simulink model "sgMdl_OPCUA_Security"  (R2024b)
settings: Solver=FixedStepAuto  StartTime=0.0  StopTime=inf  RelTol=1e-3  EnableMultiTasking=on
undefined symbols (not defined in the file): filesep, Ts
libraries: speedgoatlib_opcua x25, simulink x10
Description:
  | OPC UA Security
settings Model: sg_rtwmakecfg_data=_sg_IO75X_v1_2_0__sg_netxLib_MSVC140_  ModifiedByFormat=Speedgoat  Creator=Speedgoat  LastModifiedBy=Speedgoat
settings SolverCC: ConcurrentTasks=on  AlgebraicLoopSolver=TrustRegion  PositivePriorityOrder=on  AutoInsertRateTranBlk=on  InsertRTBMode=Never (minimum delay)  MaxZcPerStep=1
settings DataIOCC: LimitDataPoints=on  SaveFormat=StructureWithTime  ReturnWorkspaceOutputs=off
settings OptimizationCC: BlockReduction=off  BooleanDataType=off  OptimizeBlockIOStorage=off  BufferReuse=off  GlobalBufferReuse=off  ExpressionFolding=off  LocalBlockOutputs=off  OptimizeDataStoreBuffers=off  BusAssignmentInplaceUpdate=off
settings DebuggingCC: SaveWithParameterizedLinksMsg=none  UnderspecifiedInitializationDetection=Classic  MergeDetectMultiDrivingBlocksExec=none  SignalResolutionControl=TryResolveAllWithWarning  TasksWithSamePriorityMsg=none  ParameterOverflowMsg=warning  UnconnectedInputMsg=warning  UnconnectedOutputMsg=warning  UnconnectedLineMsg=warning  SFUnexpectedBacktrackingDiag=warning  SFNoUnconditionalDefaultTransitionDiag=warning  SFExecutionAtInitializationDiag=none  ArithmeticOperatorsInVariantConditions=warning
settings HardwareCC: ProdBitPerLong=64  ProdLongLongMode=on  ProdHWDeviceType=Intel->x86-64 (Linux 64)  TargetBitPerPointer=64  TargetBitPerSizeT=64  TargetBitPerPtrDiffT=64  TargetLongLongMode=on  TargetIntDivRoundTo=Zero  TargetEndianess=LittleEndian  TargetWordSize=64  TargetHWDeviceType=MATLAB Host
settings ModelReferenceCC: EnableRefExpFcnMdlSchedulingChecks=on  PropagateSignalLabelsOutOfModel=off
settings SFSimCC: SimUseLocalCustomCode=off  CustomCodeUndefinedFunction=UseInterfaceOnly
settings RTWCC: Description=Speedgoat Real-Time Target Machine  SystemTargetFile=speedgoat.tlc  TemplateMakefile=slrealtime_default_tmf  RetainRTWFile=on  RTWUseLocalCustomCode=off  Toolchain=Simulink Real-Time Toolchain  BuildConfiguration=Faster Runs  TargetLang=C++  GPUComputeCapability=3.5  DLArmComputeVersion=19.05
settings CodeAppCC: StateflowObjectComments=on
settings SimulinkRealTimeTargetCC: SubcomponentCodeInterfacePackaging=Reusable function  InstructionSetFMA=off  LogToMDFFile=off  SLRTFileLogMaxRuns=10
settings ConfigComp: CovMetricSettings=dw  CovSaveCumulativeToWorkspaceVar=on  CovSaveSingleToWorkspaceVar=on  CovExternalEMLEnable=off  CovBoundaryAbsTol=1.0e-5

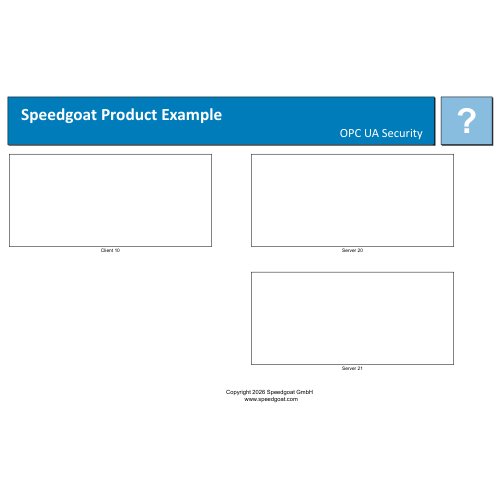
[thumbnail: Simulink's stored preview of the top-level diagram]
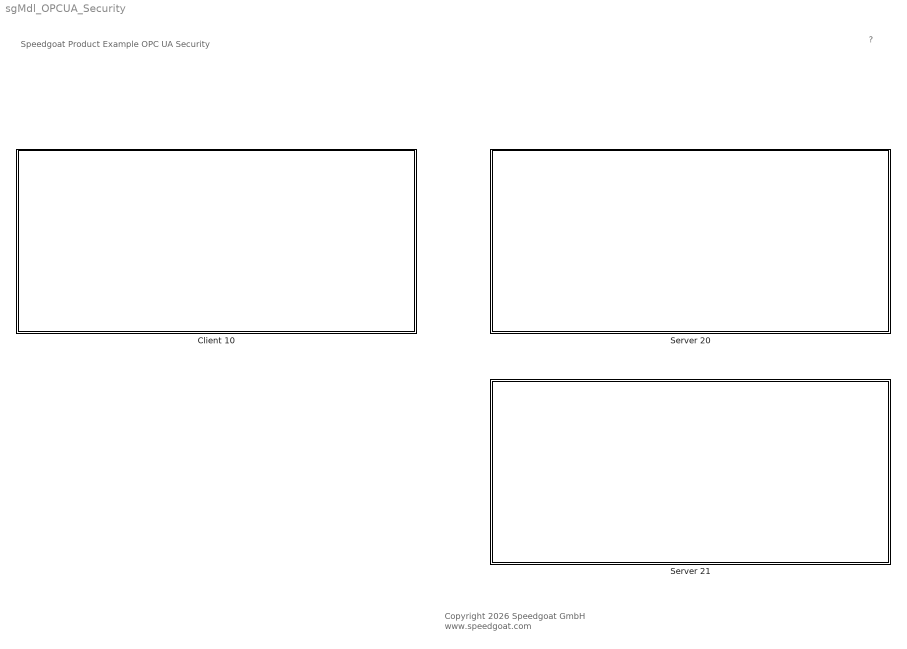
== system sgMdl_OPCUA_Security ==
  note: Speedgoat Product Example
      | OPC UA Security
  note: ?
  note: Copyright 2026 Speedgoat GmbH
      |  www.speedgoat.com
  Client 10 : Subsystem
  Server 20 : Subsystem
  Server 21 : Subsystem

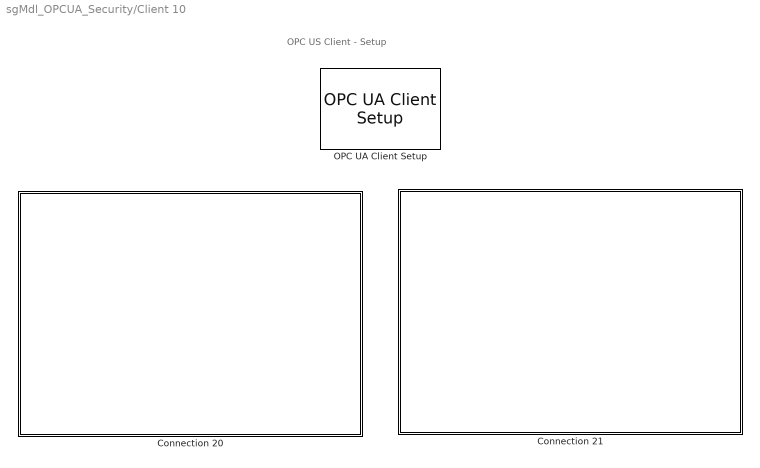
== system sgMdl_OPCUA_Security/Client 10 ==
  note: OPC US Client - Setup
  Connection 20 : Subsystem
  Connection 21 : Subsystem
  OPC UA Client Setup : speedgoatlib_opcua/Client/OPC UA Client Setup  ClientID=10  IpAddrStr=IP_Client_10
      settings: SourceProductName=OPC UA

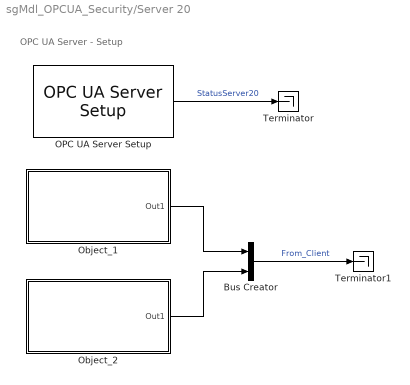
== system sgMdl_OPCUA_Security/Server 20 ==
  note: OPC UA Server - Setup
  Bus Creator : BusCreator  Inputs=2
  OPC UA Server Setup : speedgoatlib_opcua/Server/OPC UA Server Setup  ServerID=20  IpAddrStr=IP_Server_20  TcpPort=4840  NumSpaces=0  SampleTime=Ts  Endpoints={ 'None', 'on', 'None'; 'Basic128Rsa15', 'on', 'SignEncrypt'; 'Basic256', 'off', 'SignEncrypt'; 'Basic256Sha256', 'off', 'SignEncrypt'; 'Aes128_Sha256_RsaOaep', 'on', 'SignEncrypt' }  AnonymousToken=on  UsernameToken=on  Certificate=fullfile(pwd, filesep, 'cert', filesep, 'sg_server1.der')  PrivateKey=fullfile(pwd, filesep, 'cert', filesep, 'sg_key.pem')  TrustList=''  Usernames="[\"user1\", \"user2\"]"  Passwords="[\"password1\", \"password2\"]"  AppUri='urn:sg:server1'
      settings: SourceProductName=OPC UA
  Object_1 : Subsystem
  Object_2 : Subsystem
  Terminator : Terminator
  Terminator1 : Terminator
  wires:
  OPC UA Server Setup/1 -> Terminator/1  "StatusServer20"
  Object_1/1(Out1) -> Bus Creator/1
  Object_2/1(Out1) -> Bus Creator/2
  Bus Creator/1 -> Terminator1/1  "From_Client"

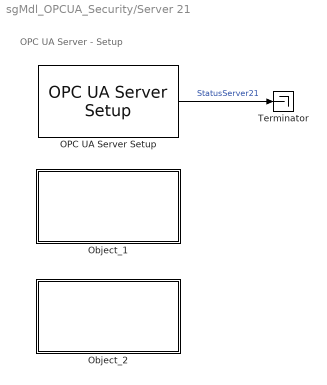
== system sgMdl_OPCUA_Security/Server 21 ==
  note: OPC UA Server - Setup
  OPC UA Server Setup : speedgoatlib_opcua/Server/OPC UA Server Setup  ServerID=21  IpAddrStr=IP_Server_21  TcpPort=4840  NumSpaces=0  SampleTime=Ts  Endpoints={ 'None', 'on', 'None'; 'Basic128Rsa15', 'off', 'SignEncrypt'; 'Basic256', 'off', 'SignEncrypt'; 'Basic256Sha256', 'on', 'SignEncrypt'; 'Aes128_Sha256_RsaOaep', 'on', 'SignEncrypt' }  AnonymousToken=off  UsernameToken=on  Certificate=fullfile(pwd, filesep, 'cert', filesep, 'sg_server2.der')  PrivateKey=fullfile(pwd, filesep, 'cert', filesep, 'sg_key.pem')  TrustList=fullfile(pwd, filesep, 'trustlist')  Usernames="[\"user1\", \"user2\"]"  Passwords="[\"password1\", \"password2\"]"  AppUri='urn:sg:server2'
      settings: SourceProductName=OPC UA
  Object_1 : Subsystem
  Object_2 : Subsystem
  Terminator : Terminator
  wires:
  OPC UA Server Setup/1 -> Terminator/1  "StatusServer21"

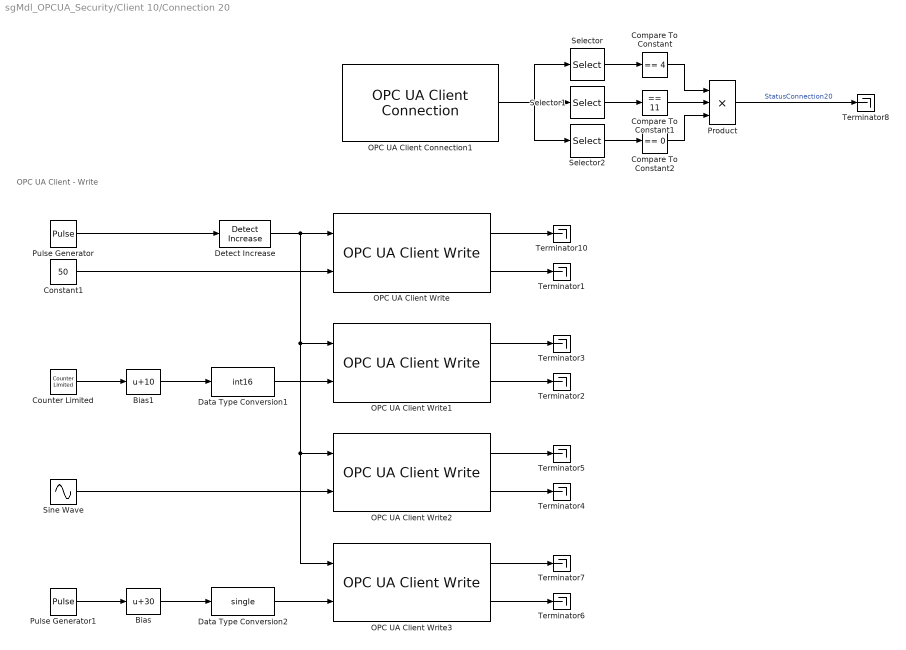
== system sgMdl_OPCUA_Security/Client 10/Connection 20 ==
  note: OPC UA Client - Write
  Bias : Bias  Bias=30  SaturateOnIntegerOverflow=off
  Bias1 : Bias  Bias=10  SaturateOnIntegerOverflow=off
  Compare To Constant : simulink/Logic and Bit Operations/Compare To Constant  relop===  const=4  OutDataTypeStr=boolean
  Compare To Constant1 : simulink/Logic and Bit Operations/Compare To Constant  relop===  const=11  OutDataTypeStr=boolean
  Compare To Constant2 : simulink/Logic and Bit Operations/Compare To Constant  relop===  const=0  OutDataTypeStr=boolean
  Constant1 : Constant  Value=50  OutDataTypeStr=int8  SampleTime=Ts
  Counter Limited : simulink/Sources/Counter Limited  uplimit=100  tsamp=0.1
  Data Type Conversion1 : DataTypeConversion  OutDataTypeStr=int16  SaturateOnIntegerOverflow=off  RndMeth=Floor
  Data Type Conversion2 : DataTypeConversion  OutDataTypeStr=single  SaturateOnIntegerOverflow=off  RndMeth=Floor
  Detect Increase : simulink/Logic and Bit Operations/Detect Increase  vinit=0.0  OutDataTypeStr=boolean
  OPC UA Client Connection1 : speedgoatlib_opcua/Client/OPC UA Client Connection  ClientID=10  ConnectionID=20  IpAddrStr=IP_Server_20  TcpPort=4840  SampleTime=Ts  SecurityPolicy=Basic128Rsa15  MessageSecurityMode=SignEncrypt  UserTokenPolicy=Username  Certificate=fullfile(pwd, filesep, 'cert', filesep, 'sg_client.der')  PrivateKey=fullfile(pwd, filesep, 'cert', filesep, 'sg_key.pem')  Username='user1'  Password='password1'  AppUri='urn:sg:client'
      settings: SourceProductName=OPC UA
  OPC UA Client Write : speedgoatlib_opcua/Client/OPC UA Client Write  ClientID=10  ConnectionID=20  StructConfig=off  Nodes=struct('Namespace',1,'IdentifierType','String','Identifier','myNode','Dimension',1,'DataType','double','SamplingInterval',500);  NodeDataType=0  NodeDimension=0  DataPortType=off  BusName='sguabus'  AddOutput=on  SampleTime=-1  Namespace=1  NodeIdType=String  NodeId='Constant'
      settings: AttributesFormatString=%<NodeId>  SourceProductName=OPC UA
  OPC UA Client Write1 : speedgoatlib_opcua/Client/OPC UA Client Write  ClientID=10  ConnectionID=20  StructConfig=off  Nodes=struct('Namespace',1,'IdentifierType','String','Identifier','myNode','Dimension',1,'DataType','double','SamplingInterval',500);  NodeDataType=0  NodeDimension=0  DataPortType=off  BusName='sguabus'  AddOutput=on  SampleTime=-1  Namespace=1  NodeIdType=String  NodeId='Counter'
      settings: AttributesFormatString=%<NodeId>  SourceProductName=OPC UA
  OPC UA Client Write2 : speedgoatlib_opcua/Client/OPC UA Client Write  ClientID=10  ConnectionID=20  StructConfig=off  Nodes=struct('Namespace',1,'IdentifierType','String','Identifier','myNode','Dimension',1,'DataType','double','SamplingInterval',500);  NodeDataType=0  NodeDimension=0  DataPortType=off  BusName='sguabus'  AddOutput=on  SampleTime=-1  Namespace=1  NodeIdType=String  NodeId='Sine'
      settings: AttributesFormatString=%<NodeId>  SourceProductName=OPC UA
  OPC UA Client Write3 : speedgoatlib_opcua/Client/OPC UA Client Write  ClientID=10  ConnectionID=20  StructConfig=off  Nodes=struct('Namespace',1,'IdentifierType','String','Identifier','myNode','Dimension',1,'DataType','double','SamplingInterval',500);  NodeDataType=0  NodeDimension=0  DataPortType=off  BusName='sguabus'  AddOutput=on  SampleTime=-1  Namespace=1  NodeIdType=String  NodeId='Pulse'
      settings: AttributesFormatString=%<NodeId>  SourceProductName=OPC UA
  Product : Product  Inputs=3
  Pulse Generator : DiscretePulseGenerator  Period=100  PulseWidth=50  SampleTime=Ts
  Pulse Generator1 : DiscretePulseGenerator  Amplitude=100  Period=4/Ts  PulseWidth=2/Ts  SampleTime=Ts
  Selector : Selector  InputPortWidth=3  IndexOptions=Index vector (dialog)  Indices=1  OutputSizes=1
  Selector1 : Selector  InputPortWidth=3  IndexOptions=Index vector (dialog)  Indices=2  OutputSizes=1
  Selector2 : Selector  InputPortWidth=3  IndexOptions=Index vector (dialog)  Indices=3  OutputSizes=1
  Sine Wave : Sin  SineType=Sample based  Amplitude=50  Bias=70  Frequency=2*pi  Phase=pi  Samples=5*1/Ts  SampleTime=Ts
  Terminator{1..8,10} (9 alike) : Terminator
  wires:
  Pulse Generator/1 -> Detect Increase/1
  Constant1/1 -> OPC UA Client Write/2
  Counter Limited/1 -> Bias1/1
  Pulse Generator1/1 -> Bias/1
  Sine Wave/1 -> OPC UA Client Write2/2
  OPC UA Client Write/1 -> Terminator10/1
  OPC UA Client Write/2 -> Terminator1/1
  Detect Increase/1 -> OPC UA Client Write2/1, OPC UA Client Write3/1, OPC UA Client Write1/1, OPC UA Client Write/1
  OPC UA Client Write1/2 -> Terminator2/1
  OPC UA Client Write1/1 -> Terminator3/1
  Data Type Conversion1/1 -> OPC UA Client Write1/2
  OPC UA Client Write3/1 -> Terminator7/1
  OPC UA Client Write3/2 -> Terminator6/1
  OPC UA Client Write2/2 -> Terminator4/1
  OPC UA Client Write2/1 -> Terminator5/1
  Data Type Conversion2/1 -> OPC UA Client Write3/2
  Compare To Constant/1 -> Product/1
  Compare To Constant2/1 -> Product/3
  Product/1 -> Terminator8/1  "StatusConnection20"
  OPC UA Client Connection1/1 -> Selector2/1, Selector/1, Selector1/1
  Compare To Constant1/1 -> Product/2
  Selector1/1 -> Compare To Constant1/1
  Selector2/1 -> Compare To Constant2/1
  Selector/1 -> Compare To Constant/1
  Bias/1 -> Data Type Conversion2/1
  Bias1/1 -> Data Type Conversion1/1

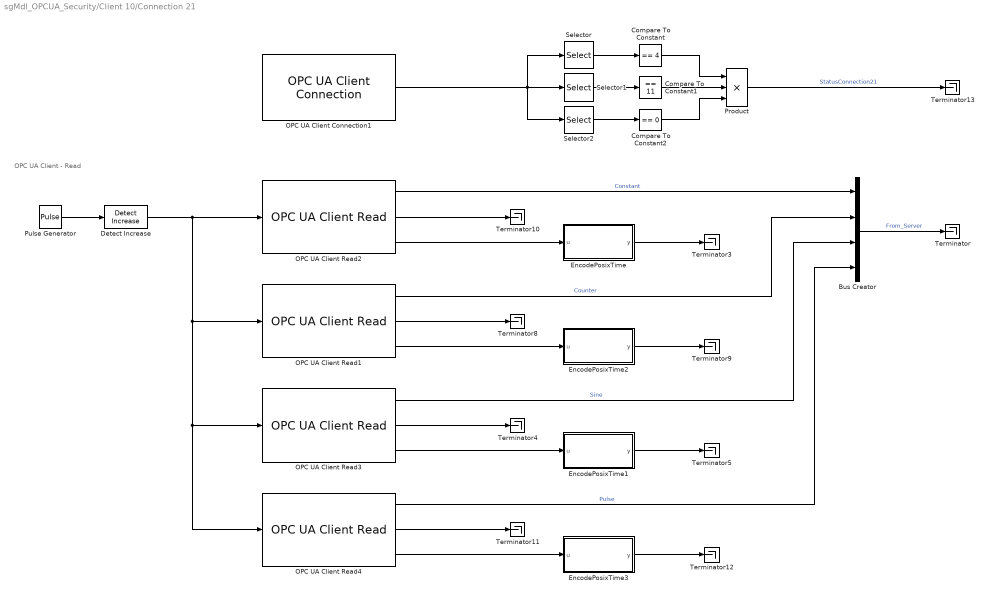
== system sgMdl_OPCUA_Security/Client 10/Connection 21 ==
  note: OPC UA Client - Read
  Bus Creator : BusCreator  Inputs=4
  Compare To Constant : simulink/Logic and Bit Operations/Compare To Constant  relop===  const=4  OutDataTypeStr=boolean
  Compare To Constant1 : simulink/Logic and Bit Operations/Compare To Constant  relop===  const=11  OutDataTypeStr=boolean
  Compare To Constant2 : simulink/Logic and Bit Operations/Compare To Constant  relop===  const=0  OutDataTypeStr=boolean
  Detect Increase : simulink/Logic and Bit Operations/Detect Increase  vinit=0.0  OutDataTypeStr=boolean
  EncodePosixTime : MATLAB Function  TreatAsAtomicUnit=on
  EncodePosixTime1 : MATLAB Function  TreatAsAtomicUnit=on
  EncodePosixTime2 : MATLAB Function  TreatAsAtomicUnit=on
  EncodePosixTime3 : MATLAB Function  TreatAsAtomicUnit=on
  OPC UA Client Connection1 : speedgoatlib_opcua/Client/OPC UA Client Connection  ClientID=10  ConnectionID=21  IpAddrStr=IP_Server_21  TcpPort=4840  SampleTime=Ts  SecurityPolicy=Basic256Sha256  MessageSecurityMode=SignEncrypt  UserTokenPolicy=Username  Certificate=fullfile(pwd, filesep, 'cert', filesep, 'sg_client.der')  PrivateKey=fullfile(pwd, filesep, 'cert', filesep, 'sg_key.pem')  Username='user2'  Password='password2'  AppUri='urn:sg:client'
      settings: SourceProductName=OPC UA
  OPC UA Client Read1 : speedgoatlib_opcua/Client/OPC UA Client Read  ClientID=10  ConnectionID=21  StructConfig=off  Nodes=struct('Namespace',1,'IdentifierType','String','Identifier','myNode','Dimension',1,'DataType','double','SamplingInterval',500);  NodeDataType=0  NodeDimension=0  DataPortType=off  BusName=0  AddOutput=on  CreateSubscription=off  SampleTime=Ts  Namespace=1  NodeIdType=String  NodeId='Counter'  InitValue=int16(0)  ForceVector=off  MonitoringMode=Reporting  SamplingInterval=500  PublishingInterval=500
      settings: AttributesFormatString=%<NodeId>  SourceProductName=OPC UA
  OPC UA Client Read2 : speedgoatlib_opcua/Client/OPC UA Client Read  ClientID=10  ConnectionID=21  StructConfig=off  Nodes=struct('Namespace',1,'IdentifierType','String','Identifier','myNode','Dimension',1,'DataType','double','SamplingInterval',500);  NodeDataType=0  NodeDimension=0  DataPortType=off  BusName=0  AddOutput=on  CreateSubscription=off  SampleTime=Ts  Namespace=1  NodeIdType=String  NodeId='Constant'  InitValue=int8(0)  ForceVector=off  MonitoringMode=Reporting  SamplingInterval=500  PublishingInterval=500
      settings: AttributesFormatString=%<NodeId>  SourceProductName=OPC UA
  OPC UA Client Read3 : speedgoatlib_opcua/Client/OPC UA Client Read  ClientID=10  ConnectionID=21  StructConfig=off  Nodes=struct('Namespace',1,'IdentifierType','String','Identifier','myNode','Dimension',1,'DataType','double','SamplingInterval',500);  NodeDataType=0  NodeDimension=0  DataPortType=off  BusName=0  AddOutput=on  CreateSubscription=off  SampleTime=Ts  Namespace=1  NodeIdType=String  NodeId='Sine'  InitValue=double(0)  ForceVector=off  MonitoringMode=Reporting  SamplingInterval=500  PublishingInterval=500
      settings: AttributesFormatString=%<NodeId>  SourceProductName=OPC UA
  OPC UA Client Read4 : speedgoatlib_opcua/Client/OPC UA Client Read  ClientID=10  ConnectionID=21  StructConfig=off  Nodes=struct('Namespace',1,'IdentifierType','String','Identifier','myNode','Dimension',1,'DataType','double','SamplingInterval',500);  NodeDataType=0  NodeDimension=0  DataPortType=off  BusName=0  AddOutput=on  CreateSubscription=off  SampleTime=Ts  Namespace=1  NodeIdType=String  NodeId='Pulse'  InitValue=single(0)  ForceVector=off  MonitoringMode=Reporting  SamplingInterval=500  PublishingInterval=500
      settings: AttributesFormatString=%<NodeId>  SourceProductName=OPC UA
  Product : Product  Inputs=3
  Pulse Generator : DiscretePulseGenerator  Period=100  PulseWidth=50  SampleTime=Ts
  Selector : Selector  InputPortWidth=3  IndexOptions=Index vector (dialog)  Indices=1  OutputSizes=1
  Selector1 : Selector  InputPortWidth=3  IndexOptions=Index vector (dialog)  Indices=2  OutputSizes=1
  Selector2 : Selector  InputPortWidth=3  IndexOptions=Index vector (dialog)  Indices=3  OutputSizes=1
  Terminator{,3..5,8..13} (10 alike) : Terminator
  wires:
  Pulse Generator/1 -> Detect Increase/1
  OPC UA Client Read2/1 -> Bus Creator/1  "Constant"
  OPC UA Client Read1/2 -> Terminator8/1
  OPC UA Client Read1/3 -> EncodePosixTime2/1(u)
  OPC UA Client Read1/1 -> Bus Creator/2  "Counter"
  EncodePosixTime2/1(y) -> Terminator9/1
  EncodePosixTime/1(y) -> Terminator3/1
  OPC UA Client Read2/2 -> Terminator10/1
  OPC UA Client Read2/3 -> EncodePosixTime/1(u)
  Detect Increase/1 -> OPC UA Client Read4/1, OPC UA Client Read3/1, OPC UA Client Read1/1, OPC UA Client Read2/1
  EncodePosixTime1/1(y) -> Terminator5/1
  OPC UA Client Read3/1 -> Bus Creator/3  "Sine"
  OPC UA Client Read3/3 -> EncodePosixTime1/1(u)
  OPC UA Client Read3/2 -> Terminator4/1
  OPC UA Client Read4/2 -> Terminator11/1
  OPC UA Client Read4/3 -> EncodePosixTime3/1(u)
  OPC UA Client Read4/1 -> Bus Creator/4  "Pulse"
  EncodePosixTime3/1(y) -> Terminator12/1
  Compare To Constant/1 -> Product/1
  Selector2/1 -> Compare To Constant2/1
  Selector1/1 -> Compare To Constant1/1
  Compare To Constant2/1 -> Product/3
  Compare To Constant1/1 -> Product/2
  Product/1 -> Terminator13/1  "StatusConnection21"
  Selector/1 -> Compare To Constant/1
  OPC UA Client Connection1/1 -> Selector2/1, Selector/1, Selector1/1
  Bus Creator/1 -> Terminator/1  "From_Server"

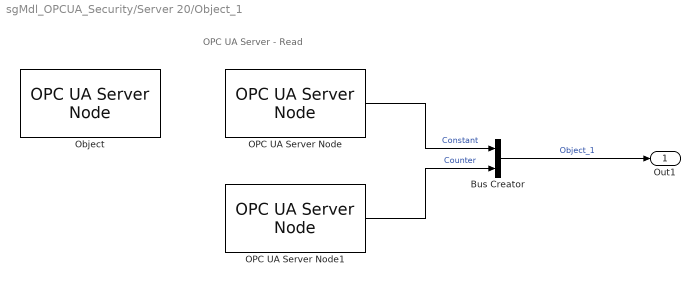
== system sgMdl_OPCUA_Security/Server 20/Object_1 ==
  note: OPC UA Server - Read
  Bus Creator : BusCreator  Inputs=2
  OPC UA Server Node : speedgoatlib_opcua/Server/OPC UA Server Node  ServerID=20  NodeType=Variable  Namespace=1  NodeIdType=String  NodeId='Constant'  ParentNodes='Object_1'  BrowseName='Constant'  DisplayName='Constant'  NodeDescription=''  InitValue=int8(0)  ForceVector=off  ReadAccess=on  WriteAccess=on  ReadOp=on  WriteOp=off  Extended=off  SampleTime=Ts
      settings: AttributesFormatString=%<NodeId>  SourceProductName=OPC UA
  OPC UA Server Node1 : speedgoatlib_opcua/Server/OPC UA Server Node  ServerID=20  NodeType=Variable  Namespace=1  NodeIdType=String  NodeId='Counter'  ParentNodes='Object_1'  BrowseName='Counter'  DisplayName='Counter'  NodeDescription=''  InitValue=int16(0)  ForceVector=off  ReadAccess=on  WriteAccess=on  ReadOp=on  WriteOp=off  Extended=off  SampleTime=Ts
      settings: AttributesFormatString=%<NodeId>  SourceProductName=OPC UA
  Object : speedgoatlib_opcua/Server/OPC UA Server Node  ServerID=20  NodeType=Object  Namespace=1  NodeIdType=String  NodeId='Object_1'  ParentNodes=''  BrowseName='Object_1'  DisplayName='Object_1'  NodeDescription=''  InitValue=[]  ForceVector=off  ReadAccess=on  WriteAccess=off  ReadOp=off  WriteOp=off  Extended=off  SampleTime=Ts
      settings: SourceProductName=OPC UA
  Out1 : Outport
  wires:
  OPC UA Server Node/1 -> Bus Creator/1  "Constant"
  OPC UA Server Node1/1 -> Bus Creator/2  "Counter"
  Bus Creator/1 -> Out1/1  "Object_1"

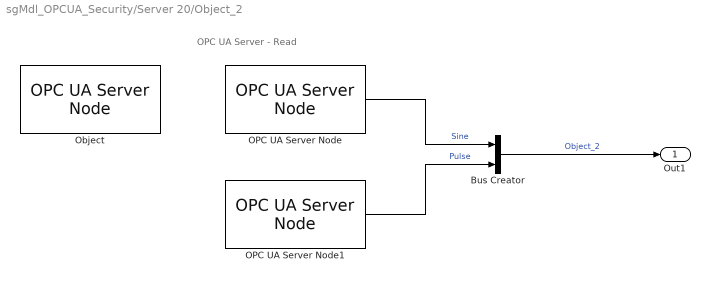
== system sgMdl_OPCUA_Security/Server 20/Object_2 ==
  note: OPC UA Server - Read
  Bus Creator : BusCreator  Inputs=2
  OPC UA Server Node : speedgoatlib_opcua/Server/OPC UA Server Node  ServerID=20  NodeType=Variable  Namespace=1  NodeIdType=String  NodeId='Sine'  ParentNodes='Object_2'  BrowseName='Sine'  DisplayName='Sine'  NodeDescription=''  InitValue=double(0)  ForceVector=off  ReadAccess=on  WriteAccess=on  ReadOp=on  WriteOp=off  Extended=off  SampleTime=Ts
      settings: AttributesFormatString=%<NodeId>  SourceProductName=OPC UA
  OPC UA Server Node1 : speedgoatlib_opcua/Server/OPC UA Server Node  ServerID=20  NodeType=Variable  Namespace=1  NodeIdType=String  NodeId='Pulse'  ParentNodes='Object_2'  BrowseName='Pulse'  DisplayName='Pulse'  NodeDescription=''  InitValue=single(0)  ForceVector=off  ReadAccess=on  WriteAccess=on  ReadOp=on  WriteOp=off  Extended=off  SampleTime=Ts
      settings: AttributesFormatString=%<NodeId>  SourceProductName=OPC UA
  Object : speedgoatlib_opcua/Server/OPC UA Server Node  ServerID=20  NodeType=Object  Namespace=1  NodeIdType=String  NodeId='Object_2'  ParentNodes=''  BrowseName='Object_2'  DisplayName='Object_2'  NodeDescription=''  InitValue=[]  ForceVector=off  ReadAccess=on  WriteAccess=off  ReadOp=off  WriteOp=off  Extended=off  SampleTime=Ts
      settings: SourceProductName=OPC UA
  Out1 : Outport
  wires:
  Bus Creator/1 -> Out1/1  "Object_2"
  OPC UA Server Node1/1 -> Bus Creator/2  "Pulse"
  OPC UA Server Node/1 -> Bus Creator/1  "Sine"

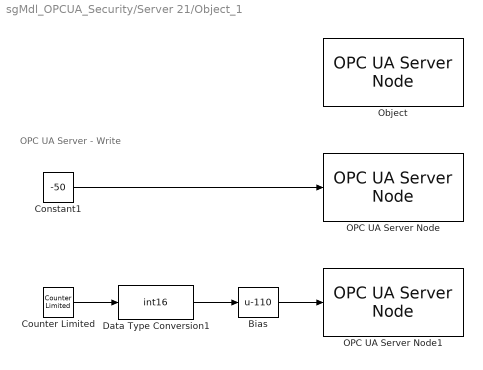
== system sgMdl_OPCUA_Security/Server 21/Object_1 ==
  note: OPC UA Server - Write
  Bias : Bias  Bias=-110  SaturateOnIntegerOverflow=off
  Constant1 : Constant  Value=-50  OutDataTypeStr=int8  SampleTime=Ts
  Counter Limited : simulink/Sources/Counter Limited  uplimit=100  tsamp=0.1
  Data Type Conversion1 : DataTypeConversion  OutDataTypeStr=int16  SaturateOnIntegerOverflow=off  RndMeth=Floor
  OPC UA Server Node : speedgoatlib_opcua/Server/OPC UA Server Node  ServerID=21  NodeType=Variable  Namespace=1  NodeIdType=String  NodeId='Constant'  ParentNodes='Object_1'  BrowseName='Constant'  DisplayName='Constant'  NodeDescription=''  InitValue=int8(0)  ForceVector=off  ReadAccess=on  WriteAccess=on  ReadOp=off  WriteOp=on  Extended=off  SampleTime=Ts
      settings: AttributesFormatString=%<NodeId>  SourceProductName=OPC UA
  OPC UA Server Node1 : speedgoatlib_opcua/Server/OPC UA Server Node  ServerID=21  NodeType=Variable  Namespace=1  NodeIdType=String  NodeId='Counter'  ParentNodes='Object_1'  BrowseName='Counter'  DisplayName='Counter'  NodeDescription=''  InitValue=int16(0)  ForceVector=off  ReadAccess=on  WriteAccess=on  ReadOp=off  WriteOp=on  Extended=off  SampleTime=Ts
      settings: AttributesFormatString=%<NodeId>  SourceProductName=OPC UA
  Object : speedgoatlib_opcua/Server/OPC UA Server Node  ServerID=21  NodeType=Object  Namespace=1  NodeIdType=String  NodeId='Object_1'  ParentNodes=''  BrowseName='Object_1'  DisplayName='Object_1'  NodeDescription=''  InitValue=[]  ForceVector=off  ReadAccess=on  WriteAccess=off  ReadOp=off  WriteOp=off  Extended=off  SampleTime=Ts
      settings: SourceProductName=OPC UA
  wires:
  Data Type Conversion1/1 -> Bias/1
  Constant1/1 -> OPC UA Server Node/1
  Counter Limited/1 -> Data Type Conversion1/1
  Bias/1 -> OPC UA Server Node1/1

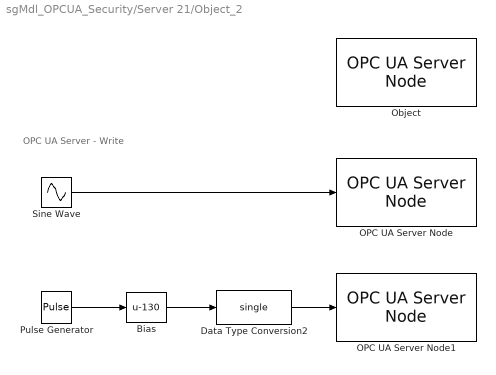
== system sgMdl_OPCUA_Security/Server 21/Object_2 ==
  note: OPC UA Server - Write
  Bias : Bias  Bias=-130  SaturateOnIntegerOverflow=off
  Data Type Conversion2 : DataTypeConversion  OutDataTypeStr=single  SaturateOnIntegerOverflow=off  RndMeth=Floor
  OPC UA Server Node : speedgoatlib_opcua/Server/OPC UA Server Node  ServerID=21  NodeType=Variable  Namespace=1  NodeIdType=String  NodeId='Sine'  ParentNodes='Object_2'  BrowseName='Sine'  DisplayName='Sine'  NodeDescription=''  InitValue=double(0)  ForceVector=off  ReadAccess=on  WriteAccess=on  ReadOp=off  WriteOp=on  Extended=off  SampleTime=Ts
      settings: AttributesFormatString=%<NodeId>  SourceProductName=OPC UA
  OPC UA Server Node1 : speedgoatlib_opcua/Server/OPC UA Server Node  ServerID=21  NodeType=Variable  Namespace=1  NodeIdType=String  NodeId='Pulse'  ParentNodes='Object_2'  BrowseName='Pulse'  DisplayName='Pulse'  NodeDescription=''  InitValue=single(0)  ForceVector=off  ReadAccess=on  WriteAccess=on  ReadOp=off  WriteOp=on  Extended=off  SampleTime=Ts
      settings: AttributesFormatString=%<NodeId>  SourceProductName=OPC UA
  Object : speedgoatlib_opcua/Server/OPC UA Server Node  ServerID=21  NodeType=Object  Namespace=1  NodeIdType=String  NodeId='Object_2'  ParentNodes=''  BrowseName='Object_2'  DisplayName='Object_2'  NodeDescription=''  InitValue=[]  ForceVector=off  ReadAccess=on  WriteAccess=off  ReadOp=off  WriteOp=off  Extended=off  SampleTime=Ts
      settings: SourceProductName=OPC UA
  Pulse Generator : DiscretePulseGenerator  Amplitude=100  Period=4*1/Ts  PulseWidth=2/Ts  SampleTime=Ts
  Sine Wave : Sin  SineType=Sample based  Amplitude=50  Bias=-70  Frequency=2*pi  Phase=pi  Samples=5*1/Ts  SampleTime=Ts
  wires:
  Sine Wave/1 -> OPC UA Server Node/1
  Pulse Generator/1 -> Bias/1
  Data Type Conversion2/1 -> OPC UA Server Node1/1
  Bias/1 -> Data Type Conversion2/1

== matlab function sgMdl_OPCUA_Security/Client 10/Connection 21/EncodePosixTime1 ==
  data: u input; y output
function y = fcn(u)

y = zeros(1,7);
y(1,1:6) = datevec(datetime(floor(u/1000),'ConvertFrom','posixtime'));
y(7) = mod(u,uint64(1000));

== matlab function sgMdl_OPCUA_Security/Client 10/Connection 21/EncodePosixTime2 ==
  data: u input; y output
function y = fcn(u)

y = zeros(1,7);
y(1,1:6) = datevec(datetime(floor(u/1000),'ConvertFrom','posixtime'));
y(7) = mod(u,uint64(1000));

== matlab function sgMdl_OPCUA_Security/Client 10/Connection 21/EncodePosixTime3 ==
  data: u input; y output
function y = fcn(u)

y = zeros(1,7);
y(1,1:6) = datevec(datetime(floor(u/1000),'ConvertFrom','posixtime'));
y(7) = mod(u,uint64(1000));

== matlab function sgMdl_OPCUA_Security/Client 10/Connection 21/EncodePosixTime ==
  data: u input; y output
function y = fcn(u)

y = zeros(1,7);
y(1,1:6) = datevec(datetime(floor(u/1000),'ConvertFrom','posixtime'));
y(7) = mod(u,uint64(1000));
